simulink model "sim_dist_pos_obs_paper"  (R2020a)
settings: Solver=ode4  StartTime=0.0  StopTime=30.0  FixedStep=0.01  RelTol=1e-3
values from neighbouring files (symbols this model uses):
  alfa_theta = 20    [draw_compare_dist_pos_obs.m]
  alfa_theta_obs = 100    [draw_compare_dist_pos_obs.m]
  beta1 = 1.2    [draw_compare_dist_pos_obs.m]
  beta2 = 0.8    [draw_compare_dist_pos_obs.m]
  c1_diff_sigma_bar_v = diag([25; 30; 20])    [draw_compare_dist_pos_obs.m]
  c1v = diag([16.0; 16.0; 16.0])    [draw_compare_dist_pos_obs.m]
  c2_diff_sigma_bar_v = diag([50; 50; 10])    [draw_compare_dist_pos_obs.m]
  c2v = diag([16.0; 16.0; 16.0])    [draw_compare_dist_pos_obs.m]
  c3_diff_sigma_bar_v = diag([15; 15; 10])    [draw_compare_dist_pos_obs.m]
  c3v = diag([16.0; 16.0; 16.0])    [draw_compare_dist_pos_obs.m]
  delta_p_i_0 = zeros(3, NF)    [draw_compare_dist_pos_obs.m]
  delta_v_i_0 = zeros(3, NF)    [draw_compare_dist_pos_obs.m]
  dp_aa_t = 0.2 * ones(3, 5) + ( 1.0 - 0.2 ) * rand(3, 5)    [draw_compare_dist_pos_obs.m]
  dp_ff_t = [ 0.4 * ones(1, 5) + ( 1.0 - 0.4 ) * rand(1, 5);                      0.4 * ones(1, 5) + ( 1.0 - 0.4 ) * rand(1, 5);                      0.2 * ones(1, 5) + ( 0.6 - 0.2 ) * rand(1, 5) ]    [draw_compare_dist_pos_obs.m]
  dp_phi_t = ( - pi / 2 ) * ones(3, 5) + ( pi / 2 - ( - pi / 2 ) ) * rand(3, 5)    [draw_compare_dist_pos_obs.m]
  etai_0 = zeros(3,5)    [draw_compare_dist_pos_obs.m]
  kai_1_t = 0.02    [draw_compare_dist_pos_obs.m]
  kai_3_t = 0.1    [draw_compare_dist_pos_obs.m]
  kai_chi_1 = diag([6; 6; 6])    [draw_compare_dist_pos_obs.m]
  kai_chi_2 = diag([6; 6; 6])    [draw_compare_dist_pos_obs.m]
  kai_u_1 = diag([8; 8; 8])    [draw_compare_dist_pos_obs.m]
  kai_u_2 = diag([8; 8; 8])    [draw_compare_dist_pos_obs.m]
  ksii_0 = zeros(3,5)    [draw_compare_dist_pos_obs.m]
  l1v = diag([20; 20; 20])    [draw_compare_dist_pos_obs.m]
  l2v = diag([30; 30; 30])    [draw_compare_dist_pos_obs.m]
  Lamd_diff_sigma_bar_v = 0.5    [draw_compare_dist_pos_obs.m]
  mass_i = zeros(1,NF)    [draw_compare_dist_pos_obs.m]
  Mii = diag([1;0;0;0;1])    [draw_compare_dist_pos_obs.m]
  pos0 = zeros(3, 1)    [draw_compare_dist_pos_obs.m]
  PZ0 = P0(3)    [draw_compare_dist_pos_obs.m]
  PZ1 = 10    [draw_compare_dist_pos_obs.m]
  Qci_init = repmat([1;0;0;0],1,NF)    [draw_compare_dist_pos_obs.m]
  R0 = 4    [draw_compare_dist_pos_obs.m]
  R1 = 8    [draw_compare_dist_pos_obs.m]
  Rx2 = 10    [draw_compare_dist_pos_obs.m]
  Ry2 = 6    [draw_compare_dist_pos_obs.m]
  Rz2 = 4    [draw_compare_dist_pos_obs.m]
  T0 = 0    [draw_compare_dist_pos_obs.m]
  T1 = tseq1    (= 10)    [draw_compare_dist_pos_obs.m]
  T12 = tseq1 + tseq12    (= 20)    [draw_compare_dist_pos_obs.m]
  T2 = tseq1 + tseq12 + tseq2    (= 30)    [draw_compare_dist_pos_obs.m]
  theta0 = ( 2 / 5 ) * pi    (= 1.25663706144)    [draw_compare_dist_pos_obs.m]
  vel0 = zeros(3, 1)    [draw_compare_dist_pos_obs.m]
  Wij = [0,0,1,0,0;              0,0,1,1,0;              1,0,0,0,1;              0,1,1,0,0;              0,0,1,0,0]    [draw_compare_dist_pos_obs.m]
  X1 = 8    [draw_compare_dist_pos_obs.m]
  X2 = 2    [draw_compare_dist_pos_obs.m]
  X3 = 3    [draw_compare_dist_pos_obs.m]
  Y1 = 10    [draw_compare_dist_pos_obs.m]
  Y2 = 2    [draw_compare_dist_pos_obs.m]
  Y3 = 4    [draw_compare_dist_pos_obs.m]
  Z1 = 4    [draw_compare_dist_pos_obs.m]
  Z2 = -6    [draw_compare_dist_pos_obs.m]
  Z3 = 2    [draw_compare_dist_pos_obs.m]
  zeta_diff_sigma_bar_v = 0.08    [draw_compare_dist_pos_obs.m]
undefined symbols (not defined in the file or in its folder): cal_frac_squ, p_alfav1, p_alfav2, p_beta1, p_beta2, p_dbeta1, p_dbeta2, p_gamma1_pos, p_gamma1_vel, p_gamma2_pos, p_gamma2_vel, q_alfav1, q_alfav2, q_beta1, q_beta2, q_dbeta1, q_dbeta2, q_gamma1_pos, q_gamma1_vel, q_gamma2_pos, q_gamma2_vel
(part 2 of 5)

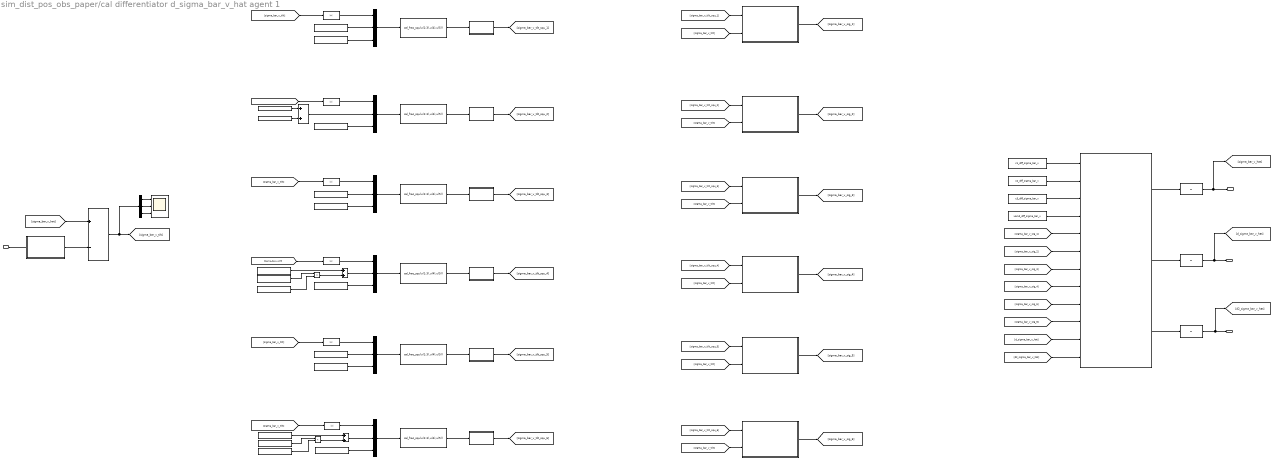
== system sim_dist_pos_obs_paper/cal differentiator d_sigma_bar_v_hat agent 1 ==
  x : Inport
  Abs{,1..5} (6 alike) : Abs
  Add : Sum
  Add1 : Sum
  Add2 : Sum
  Add3 : Sum  Inputs=+-
  Constant : Constant  Value=0
  Constant{97,100,105,107,109} (5 alike) : Constant
  Constant{98..99,101,108,110..111} (6 alike) : Constant  Value=3
  Constant102 : Constant  Value=2
  Constant103 : Constant  Value=c1_diff_sigma_bar_v
  Constant104 : Constant  Value=c2_diff_sigma_bar_v
  Constant106 : Constant  Value=c3_diff_sigma_bar_v
  Constant112 : Constant  Value=2
  Constant113 : Constant  Value=Lamd_diff_sigma_bar_v
  Constant161 : Constant  Value=zeta_diff_sigma_bar_v
  Constant162 : Constant  Value=zeta_diff_sigma_bar_v
  Constant163 : Constant  Value=zeta_diff_sigma_bar_v
  Demux2 : Demux  Outputs=3
  Integrator2 : Integrator  InitialCondition=zeros(3,1)
  Integrator3 : Integrator  InitialCondition=zeros(3,1)
  Integrator4 : Integrator  InitialCondition=zeros(3,1)
  Interpreted MATLAB Function{,20..24} (6 alike) : MATLABFcn  MATLABFcn=cal_frac_squ(u(1:3),u(4),u(5))
  Mux{19..24} (6 alike) : Mux  Inputs=3
  Product : Product
  Product1 : Product
  cal differentiator : MATLAB Function  TreatAsAtomicUnit=on
  cal sig : MATLAB Function  TreatAsAtomicUnit=on
  cal sig1 : MATLAB Function  TreatAsAtomicUnit=on
  cal sig2 : MATLAB Function  TreatAsAtomicUnit=on
  cal sig3 : MATLAB Function  TreatAsAtomicUnit=on
  cal sig4 : MATLAB Function  TreatAsAtomicUnit=on
  cal sig5 : MATLAB Function  TreatAsAtomicUnit=on
  choose sigma_bar_v : MATLAB Function  TreatAsAtomicUnit=on
  sigma_bar_v_tilt : Scope  NumInputPorts=3
  trans to column20 : MATLAB Function  TreatAsAtomicUnit=on
  trans to column21 : MATLAB Function  TreatAsAtomicUnit=on
  trans to column22 : MATLAB Function  TreatAsAtomicUnit=on
  trans to column23 : MATLAB Function  TreatAsAtomicUnit=on
  trans to column24 : MATLAB Function  TreatAsAtomicUnit=on
  trans to column25 : MATLAB Function  TreatAsAtomicUnit=on
  Out1 : Outport
  Out2 : Outport  Port=2
  Out3 : Outport  Port=3
  wires:
  Abs/1 -> Mux22/1
  [sigma_bar_v_tilt] -> cal sig/2(y)
  cal sig1/1(z) -> [sigma_bar_v_sig_2]
  [d2_sigma_bar_v_hat] -> cal differentiator/12(d2_sigma_bar_v_hat)
  trans to column23/1(y) -> [sigma_bar_v_tilt_squ_3]
  Add/1 -> Mux21/2
  Demux2/1 -> sigma_bar_v_tilt/1
  [sigma_bar_v_tilt] -> cal sig4/2(y)
  Product1/1 -> Add2/2
  Add2/1 -> Mux19/2
  [d_sigma_bar_v_hat] -> cal differentiator/11("d_sigma_bar_v_hat ")
  [sigma_bar_v_sig_3] -> cal differentiator/7(sigma_bar_v_sig_3)
  trans to column24/1(y) -> [sigma_bar_v_tilt_squ_4]
  Constant107/1 -> Mux21/3
  [sigma_bar_v_sig_5] -> cal differentiator/9(sigma_bar_v_sig_5)
  Constant97/1 -> Mux22/3
  cal sig/1(z) -> [sigma_bar_v_sig_1]
  trans to column22/1(y) -> [sigma_bar_v_tilt_squ_1]
  [sigma_bar_v_tilt_squ_3] -> cal sig2/1(x)
  [sigma_bar_v_tilt] -> Abs3/1
  Interpreted MATLAB Function24/1 -> trans to column25/1(x)
  [sigma_bar_v_sig_1] -> cal differentiator/5(sigma_bar_v_sig_1)
  cal differentiator/1(d_sigma_bar_v_hat) -> Integrator2/1
  Constant110/1 -> Mux24/3
  cal sig5/1(z) -> [sigma_bar_v_sig_5]
  [sigma_bar_v_tilt] -> Abs4/1
  Demux2/3 -> sigma_bar_v_tilt/3
  cal sig2/1(z) -> [sigma_bar_v_sig_3]
  Constant112/1 -> Product/1
  Constant/1 -> Mux22/2
  cal differentiator/3(d_d2sigma_bar_v_hat) -> Integrator4/1
  Abs3/1 -> Mux24/1
  trans to column21/1(y) -> [sigma_bar_v_tilt_squ_2]
  Constant99/1 -> Add2/1
  Constant103/1 -> cal differentiator/1(c1)
  Mux19/1 -> Interpreted MATLAB Function24/1
  [sigma_bar_v_tilt_squ_6] -> cal sig3/1(x)
  Constant106/1 -> cal differentiator/3(c3)
  [sigma_bar_v_tilt] -> Abs2/1
  [sigma_bar_v_tilt_squ_2] -> cal sig1/1(x)
  Constant162/1 -> Product/2
  Product/1 -> Add1/2
  [sigma_bar_v_sig_4] -> cal differentiator/8(sigma_bar_v_sig_4)
  [sigma_bar_v_hat] -> Add3/1
  Constant102/1 -> Mux20/2
  Add3/1 -> Demux2/1, [sigma_bar_v_tilt]
  cal differentiator/2(d_dsigma_bar_v_hat) -> Integrator3/1
  [sigma_bar_v_tilt] -> Abs5/1
  [sigma_bar_v_tilt] -> cal sig2/2(y)
  [sigma_bar_v_sig_6] -> cal differentiator/10(sigma_bar_v_sig_6)
  trans to column20/1(y) -> [sigma_bar_v_tilt_squ_5]
  Constant104/1 -> cal differentiator/2(c2)
  Constant101/1 -> Mux20/3
  Mux22/1 -> Interpreted MATLAB Function/1
  Constant163/1 -> Product1/2
  Abs2/1 -> Mux23/1
  Interpreted MATLAB Function21/1 -> trans to column21/1(x)
  Interpreted MATLAB Function23/1 -> trans to column24/1(x)
  Mux23/1 -> Interpreted MATLAB Function22/1
  cal sig3/1(z) -> [sigma_bar_v_sig_6]
  Abs4/1 -> Mux19/1
  trans to column25/1(y) -> [sigma_bar_v_tilt_squ_6]
  Constant113/1 -> cal differentiator/4(chi_t)
  choose sigma_bar_v/1(y) -> Add3/2
  Interpreted MATLAB Function/1 -> trans to column22/1(x)
  Interpreted MATLAB Function20/1 -> trans to column20/1(x)
  Constant108/1 -> Mux23/3
  [sigma_bar_v_sig_2] -> cal differentiator/6(sigma_bar_v_sig_2)
  [sigma_bar_v_tilt] -> cal sig1/2(y)
  [sigma_bar_v_tilt_squ_1] -> cal sig/1(x)
  Constant100/1 -> Product1/1
  Abs1/1 -> Mux21/1
  Demux2/2 -> sigma_bar_v_tilt/2
  Integrator4/1 -> [d2_sigma_bar_v_hat], Out3/1
  [sigma_bar_v_tilt_squ_4] -> cal sig4/1(x)
  Abs5/1 -> Mux20/1
  Constant98/1 -> Mux19/3
  Constant111/1 -> Add1/1
  [sigma_bar_v_tilt] -> cal sig5/2(y)
  Constant109/1 -> Mux23/2
  [sigma_bar_v_tilt] -> Abs/1
  Mux24/1 -> Interpreted MATLAB Function23/1
  [sigma_bar_v_tilt] -> Abs1/1
  [sigma_bar_v_tilt_squ_5] -> cal sig5/1(x)
  Add1/1 -> Mux24/2
  cal sig4/1(z) -> [sigma_bar_v_sig_4]
  Constant161/1 -> Add/2
  [sigma_bar_v_tilt] -> cal sig3/2(y)
  Mux21/1 -> Interpreted MATLAB Function21/1
  Interpreted MATLAB Function22/1 -> trans to column23/1(x)
  Mux20/1 -> Interpreted MATLAB Function20/1
  x/1 -> choose sigma_bar_v/1(x)
  Constant105/1 -> Add/1
  Integrator2/1 -> [sigma_bar_v_hat], Out1/1
  Integrator3/1 -> [d_sigma_bar_v_hat], Out2/1

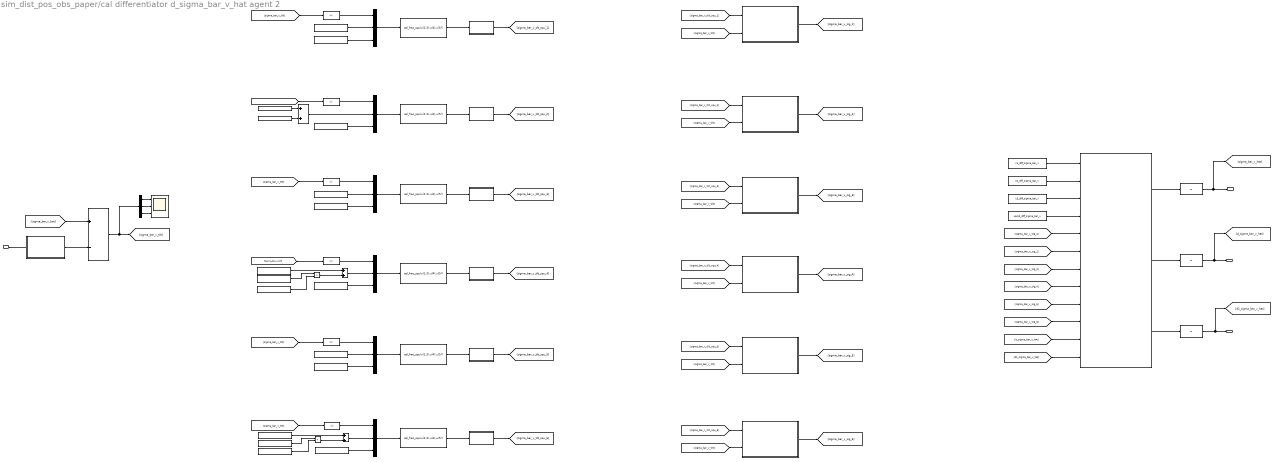
== system sim_dist_pos_obs_paper/cal differentiator d_sigma_bar_v_hat agent 2 ==
  x : Inport
  Abs{,1..5} (6 alike) : Abs
  Add : Sum
  Add1 : Sum
  Add2 : Sum
  Add3 : Sum  Inputs=+-
  Constant : Constant  Value=0
  Constant{97,100,105,107,109} (5 alike) : Constant
  Constant{98..99,101,108,110..111} (6 alike) : Constant  Value=3
  Constant102 : Constant  Value=2
  Constant103 : Constant  Value=c1_diff_sigma_bar_v
  Constant104 : Constant  Value=c2_diff_sigma_bar_v
  Constant106 : Constant  Value=c3_diff_sigma_bar_v
  Constant112 : Constant  Value=2
  Constant113 : Constant  Value=Lamd_diff_sigma_bar_v
  Constant161 : Constant  Value=zeta_diff_sigma_bar_v
  Constant162 : Constant  Value=zeta_diff_sigma_bar_v
  Constant163 : Constant  Value=zeta_diff_sigma_bar_v
  Demux2 : Demux  Outputs=3
  Integrator2 : Integrator  InitialCondition=zeros(3,1)
  Integrator3 : Integrator  InitialCondition=zeros(3,1)
  Integrator4 : Integrator  InitialCondition=zeros(3,1)
  Interpreted MATLAB Function{,20..24} (6 alike) : MATLABFcn  MATLABFcn=cal_frac_squ(u(1:3),u(4),u(5))
  Mux{19..24} (6 alike) : Mux  Inputs=3
  Product : Product
  Product1 : Product
  cal differentiator : MATLAB Function  TreatAsAtomicUnit=on
  cal sig : MATLAB Function  TreatAsAtomicUnit=on
  cal sig1 : MATLAB Function  TreatAsAtomicUnit=on
  cal sig2 : MATLAB Function  TreatAsAtomicUnit=on
  cal sig3 : MATLAB Function  TreatAsAtomicUnit=on
  cal sig4 : MATLAB Function  TreatAsAtomicUnit=on
  cal sig5 : MATLAB Function  TreatAsAtomicUnit=on
  choose sigma_bar_v : MATLAB Function  TreatAsAtomicUnit=on
  sigma_bar_v_tilt : Scope  NumInputPorts=3
  trans to column20 : MATLAB Function  TreatAsAtomicUnit=on
  trans to column21 : MATLAB Function  TreatAsAtomicUnit=on
  trans to column22 : MATLAB Function  TreatAsAtomicUnit=on
  trans to column23 : MATLAB Function  TreatAsAtomicUnit=on
  trans to column24 : MATLAB Function  TreatAsAtomicUnit=on
  trans to column25 : MATLAB Function  TreatAsAtomicUnit=on
  Out1 : Outport
  Out2 : Outport  Port=2
  Out3 : Outport  Port=3
  wires:
  Abs/1 -> Mux22/1
  [sigma_bar_v_tilt] -> cal sig/2(y)
  cal sig1/1(z) -> [sigma_bar_v_sig_2]
  [d2_sigma_bar_v_hat] -> cal differentiator/12(d2_sigma_bar_v_hat)
  trans to column23/1(y) -> [sigma_bar_v_tilt_squ_3]
  Add/1 -> Mux21/2
  Demux2/1 -> sigma_bar_v_tilt/1
  [sigma_bar_v_tilt] -> cal sig4/2(y)
  Product1/1 -> Add2/2
  Add2/1 -> Mux19/2
  [d_sigma_bar_v_hat] -> cal differentiator/11("d_sigma_bar_v_hat ")
  [sigma_bar_v_sig_3] -> cal differentiator/7(sigma_bar_v_sig_3)
  trans to column24/1(y) -> [sigma_bar_v_tilt_squ_4]
  Constant107/1 -> Mux21/3
  [sigma_bar_v_sig_5] -> cal differentiator/9(sigma_bar_v_sig_5)
  Constant97/1 -> Mux22/3
  cal sig/1(z) -> [sigma_bar_v_sig_1]
  trans to column22/1(y) -> [sigma_bar_v_tilt_squ_1]
  [sigma_bar_v_tilt_squ_3] -> cal sig2/1(x)
  [sigma_bar_v_tilt] -> Abs3/1
  Interpreted MATLAB Function24/1 -> trans to column25/1(x)
  [sigma_bar_v_sig_1] -> cal differentiator/5(sigma_bar_v_sig_1)
  cal differentiator/1(d_sigma_bar_v_hat) -> Integrator2/1
  Constant110/1 -> Mux24/3
  cal sig5/1(z) -> [sigma_bar_v_sig_5]
  [sigma_bar_v_tilt] -> Abs4/1
  Demux2/3 -> sigma_bar_v_tilt/3
  cal sig2/1(z) -> [sigma_bar_v_sig_3]
  Constant112/1 -> Product/1
  Constant/1 -> Mux22/2
  cal differentiator/3(d_d2sigma_bar_v_hat) -> Integrator4/1
  Abs3/1 -> Mux24/1
  trans to column21/1(y) -> [sigma_bar_v_tilt_squ_2]
  Constant99/1 -> Add2/1
  Constant103/1 -> cal differentiator/1(c1)
  Mux19/1 -> Interpreted MATLAB Function24/1
  [sigma_bar_v_tilt_squ_6] -> cal sig3/1(x)
  Constant106/1 -> cal differentiator/3(c3)
  [sigma_bar_v_tilt] -> Abs2/1
  [sigma_bar_v_tilt_squ_2] -> cal sig1/1(x)
  Constant162/1 -> Product/2
  Product/1 -> Add1/2
  [sigma_bar_v_sig_4] -> cal differentiator/8(sigma_bar_v_sig_4)
  [sigma_bar_v_hat] -> Add3/1
  Constant102/1 -> Mux20/2
  Add3/1 -> Demux2/1, [sigma_bar_v_tilt]
  cal differentiator/2(d_dsigma_bar_v_hat) -> Integrator3/1
  [sigma_bar_v_tilt] -> Abs5/1
  [sigma_bar_v_tilt] -> cal sig2/2(y)
  [sigma_bar_v_sig_6] -> cal differentiator/10(sigma_bar_v_sig_6)
  trans to column20/1(y) -> [sigma_bar_v_tilt_squ_5]
  Constant104/1 -> cal differentiator/2(c2)
  Constant101/1 -> Mux20/3
  Mux22/1 -> Interpreted MATLAB Function/1
  Constant163/1 -> Product1/2
  Abs2/1 -> Mux23/1
  Interpreted MATLAB Function21/1 -> trans to column21/1(x)
  Interpreted MATLAB Function23/1 -> trans to column24/1(x)
  Mux23/1 -> Interpreted MATLAB Function22/1
  cal sig3/1(z) -> [sigma_bar_v_sig_6]
  Abs4/1 -> Mux19/1
  trans to column25/1(y) -> [sigma_bar_v_tilt_squ_6]
  Constant113/1 -> cal differentiator/4(chi_t)
  choose sigma_bar_v/1(y) -> Add3/2
  Interpreted MATLAB Function/1 -> trans to column22/1(x)
  Interpreted MATLAB Function20/1 -> trans to column20/1(x)
  Constant108/1 -> Mux23/3
  [sigma_bar_v_sig_2] -> cal differentiator/6(sigma_bar_v_sig_2)
  [sigma_bar_v_tilt] -> cal sig1/2(y)
  [sigma_bar_v_tilt_squ_1] -> cal sig/1(x)
  Constant100/1 -> Product1/1
  Abs1/1 -> Mux21/1
  Demux2/2 -> sigma_bar_v_tilt/2
  Integrator4/1 -> [d2_sigma_bar_v_hat], Out3/1
  [sigma_bar_v_tilt_squ_4] -> cal sig4/1(x)
  Abs5/1 -> Mux20/1
  Constant98/1 -> Mux19/3
  Constant111/1 -> Add1/1
  [sigma_bar_v_tilt] -> cal sig5/2(y)
  Constant109/1 -> Mux23/2
  [sigma_bar_v_tilt] -> Abs/1
  Mux24/1 -> Interpreted MATLAB Function23/1
  [sigma_bar_v_tilt] -> Abs1/1
  [sigma_bar_v_tilt_squ_5] -> cal sig5/1(x)
  Add1/1 -> Mux24/2
  cal sig4/1(z) -> [sigma_bar_v_sig_4]
  Constant161/1 -> Add/2
  [sigma_bar_v_tilt] -> cal sig3/2(y)
  Mux21/1 -> Interpreted MATLAB Function21/1
  Interpreted MATLAB Function22/1 -> trans to column23/1(x)
  Mux20/1 -> Interpreted MATLAB Function20/1
  x/1 -> choose sigma_bar_v/1(x)
  Constant105/1 -> Add/1
  Integrator2/1 -> [sigma_bar_v_hat], Out1/1
  Integrator3/1 -> [d_sigma_bar_v_hat], Out2/1

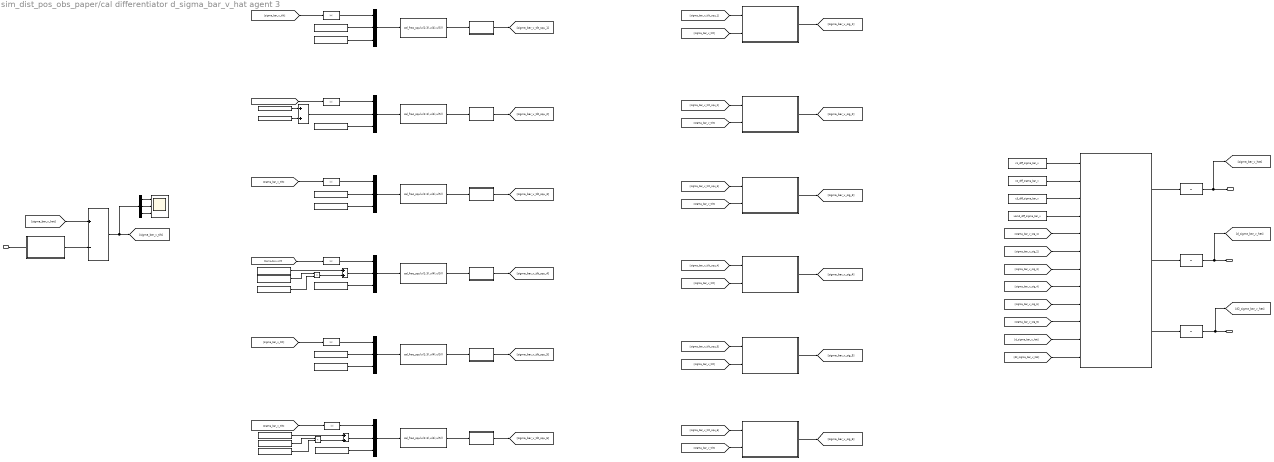
== system sim_dist_pos_obs_paper/cal differentiator d_sigma_bar_v_hat agent 3 ==
  x : Inport
  Abs{,1..5} (6 alike) : Abs
  Add : Sum
  Add1 : Sum
  Add2 : Sum
  Add3 : Sum  Inputs=+-
  Constant : Constant  Value=0
  Constant{97,100,105,107,109} (5 alike) : Constant
  Constant{98..99,101,108,110..111} (6 alike) : Constant  Value=3
  Constant102 : Constant  Value=2
  Constant103 : Constant  Value=c1_diff_sigma_bar_v
  Constant104 : Constant  Value=c2_diff_sigma_bar_v
  Constant106 : Constant  Value=c3_diff_sigma_bar_v
  Constant112 : Constant  Value=2
  Constant113 : Constant  Value=Lamd_diff_sigma_bar_v
  Constant161 : Constant  Value=zeta_diff_sigma_bar_v
  Constant162 : Constant  Value=zeta_diff_sigma_bar_v
  Constant163 : Constant  Value=zeta_diff_sigma_bar_v
  Demux2 : Demux  Outputs=3
  Integrator2 : Integrator  InitialCondition=zeros(3,1)
  Integrator3 : Integrator  InitialCondition=zeros(3,1)
  Integrator4 : Integrator  InitialCondition=zeros(3,1)
  Interpreted MATLAB Function{,20..24} (6 alike) : MATLABFcn  MATLABFcn=cal_frac_squ(u(1:3),u(4),u(5))
  Mux{19..24} (6 alike) : Mux  Inputs=3
  Product : Product
  Product1 : Product
  cal differentiator : MATLAB Function  TreatAsAtomicUnit=on
  cal sig : MATLAB Function  TreatAsAtomicUnit=on
  cal sig1 : MATLAB Function  TreatAsAtomicUnit=on
  cal sig2 : MATLAB Function  TreatAsAtomicUnit=on
  cal sig3 : MATLAB Function  TreatAsAtomicUnit=on
  cal sig4 : MATLAB Function  TreatAsAtomicUnit=on
  cal sig5 : MATLAB Function  TreatAsAtomicUnit=on
  choose sigma_bar_v : MATLAB Function  TreatAsAtomicUnit=on
  sigma_bar_v_tilt : Scope  NumInputPorts=3
  trans to column20 : MATLAB Function  TreatAsAtomicUnit=on
  trans to column21 : MATLAB Function  TreatAsAtomicUnit=on
  trans to column22 : MATLAB Function  TreatAsAtomicUnit=on
  trans to column23 : MATLAB Function  TreatAsAtomicUnit=on
  trans to column24 : MATLAB Function  TreatAsAtomicUnit=on
  trans to column25 : MATLAB Function  TreatAsAtomicUnit=on
  Out1 : Outport
  Out2 : Outport  Port=2
  Out3 : Outport  Port=3
  wires:
  Abs/1 -> Mux22/1
  [sigma_bar_v_tilt] -> cal sig/2(y)
  cal sig1/1(z) -> [sigma_bar_v_sig_2]
  [d2_sigma_bar_v_hat] -> cal differentiator/12(d2_sigma_bar_v_hat)
  trans to column23/1(y) -> [sigma_bar_v_tilt_squ_3]
  Add/1 -> Mux21/2
  Demux2/1 -> sigma_bar_v_tilt/1
  [sigma_bar_v_tilt] -> cal sig4/2(y)
  Product1/1 -> Add2/2
  Add2/1 -> Mux19/2
  [d_sigma_bar_v_hat] -> cal differentiator/11("d_sigma_bar_v_hat ")
  [sigma_bar_v_sig_3] -> cal differentiator/7(sigma_bar_v_sig_3)
  trans to column24/1(y) -> [sigma_bar_v_tilt_squ_4]
  Constant107/1 -> Mux21/3
  [sigma_bar_v_sig_5] -> cal differentiator/9(sigma_bar_v_sig_5)
  Constant97/1 -> Mux22/3
  cal sig/1(z) -> [sigma_bar_v_sig_1]
  trans to column22/1(y) -> [sigma_bar_v_tilt_squ_1]
  [sigma_bar_v_tilt_squ_3] -> cal sig2/1(x)
  [sigma_bar_v_tilt] -> Abs3/1
  Interpreted MATLAB Function24/1 -> trans to column25/1(x)
  [sigma_bar_v_sig_1] -> cal differentiator/5(sigma_bar_v_sig_1)
  cal differentiator/1(d_sigma_bar_v_hat) -> Integrator2/1
  Constant110/1 -> Mux24/3
  cal sig5/1(z) -> [sigma_bar_v_sig_5]
  [sigma_bar_v_tilt] -> Abs4/1
  Demux2/3 -> sigma_bar_v_tilt/3
  cal sig2/1(z) -> [sigma_bar_v_sig_3]
  Constant112/1 -> Product/1
  Constant/1 -> Mux22/2
  cal differentiator/3(d_d2sigma_bar_v_hat) -> Integrator4/1
  Abs3/1 -> Mux24/1
  trans to column21/1(y) -> [sigma_bar_v_tilt_squ_2]
  Constant99/1 -> Add2/1
  Constant103/1 -> cal differentiator/1(c1)
  Mux19/1 -> Interpreted MATLAB Function24/1
  [sigma_bar_v_tilt_squ_6] -> cal sig3/1(x)
  Constant106/1 -> cal differentiator/3(c3)
  [sigma_bar_v_tilt] -> Abs2/1
  [sigma_bar_v_tilt_squ_2] -> cal sig1/1(x)
  Constant162/1 -> Product/2
  Product/1 -> Add1/2
  [sigma_bar_v_sig_4] -> cal differentiator/8(sigma_bar_v_sig_4)
  [sigma_bar_v_hat] -> Add3/1
  Constant102/1 -> Mux20/2
  Add3/1 -> Demux2/1, [sigma_bar_v_tilt]
  cal differentiator/2(d_dsigma_bar_v_hat) -> Integrator3/1
  [sigma_bar_v_tilt] -> Abs5/1
  [sigma_bar_v_tilt] -> cal sig2/2(y)
  [sigma_bar_v_sig_6] -> cal differentiator/10(sigma_bar_v_sig_6)
  trans to column20/1(y) -> [sigma_bar_v_tilt_squ_5]
  Constant104/1 -> cal differentiator/2(c2)
  Constant101/1 -> Mux20/3
  Mux22/1 -> Interpreted MATLAB Function/1
  Constant163/1 -> Product1/2
  Abs2/1 -> Mux23/1
  Interpreted MATLAB Function21/1 -> trans to column21/1(x)
  Interpreted MATLAB Function23/1 -> trans to column24/1(x)
  Mux23/1 -> Interpreted MATLAB Function22/1
  cal sig3/1(z) -> [sigma_bar_v_sig_6]
  Abs4/1 -> Mux19/1
  trans to column25/1(y) -> [sigma_bar_v_tilt_squ_6]
  Constant113/1 -> cal differentiator/4(chi_t)
  choose sigma_bar_v/1(y) -> Add3/2
  Interpreted MATLAB Function/1 -> trans to column22/1(x)
  Interpreted MATLAB Function20/1 -> trans to column20/1(x)
  Constant108/1 -> Mux23/3
  [sigma_bar_v_sig_2] -> cal differentiator/6(sigma_bar_v_sig_2)
  [sigma_bar_v_tilt] -> cal sig1/2(y)
  [sigma_bar_v_tilt_squ_1] -> cal sig/1(x)
  Constant100/1 -> Product1/1
  Abs1/1 -> Mux21/1
  Demux2/2 -> sigma_bar_v_tilt/2
  Integrator4/1 -> [d2_sigma_bar_v_hat], Out3/1
  [sigma_bar_v_tilt_squ_4] -> cal sig4/1(x)
  Abs5/1 -> Mux20/1
  Constant98/1 -> Mux19/3
  Constant111/1 -> Add1/1
  [sigma_bar_v_tilt] -> cal sig5/2(y)
  Constant109/1 -> Mux23/2
  [sigma_bar_v_tilt] -> Abs/1
  Mux24/1 -> Interpreted MATLAB Function23/1
  [sigma_bar_v_tilt] -> Abs1/1
  [sigma_bar_v_tilt_squ_5] -> cal sig5/1(x)
  Add1/1 -> Mux24/2
  cal sig4/1(z) -> [sigma_bar_v_sig_4]
  Constant161/1 -> Add/2
  [sigma_bar_v_tilt] -> cal sig3/2(y)
  Mux21/1 -> Interpreted MATLAB Function21/1
  Interpreted MATLAB Function22/1 -> trans to column23/1(x)
  Mux20/1 -> Interpreted MATLAB Function20/1
  x/1 -> choose sigma_bar_v/1(x)
  Constant105/1 -> Add/1
  Integrator2/1 -> [sigma_bar_v_hat], Out1/1
  Integrator3/1 -> [d_sigma_bar_v_hat], Out2/1

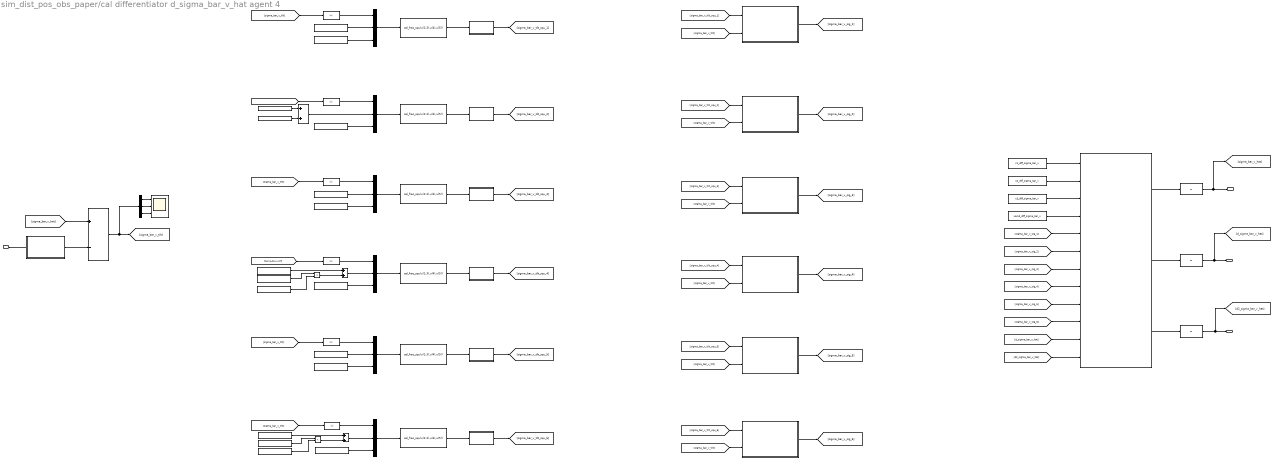
== system sim_dist_pos_obs_paper/cal differentiator d_sigma_bar_v_hat agent 4 ==
  x : Inport
  Abs{,1..5} (6 alike) : Abs
  Add : Sum
  Add1 : Sum
  Add2 : Sum
  Add3 : Sum  Inputs=+-
  Constant : Constant  Value=0
  Constant{97,100,105,107,109} (5 alike) : Constant
  Constant{98..99,101,108,110..111} (6 alike) : Constant  Value=3
  Constant102 : Constant  Value=2
  Constant103 : Constant  Value=c1_diff_sigma_bar_v
  Constant104 : Constant  Value=c2_diff_sigma_bar_v
  Constant106 : Constant  Value=c3_diff_sigma_bar_v
  Constant112 : Constant  Value=2
  Constant113 : Constant  Value=Lamd_diff_sigma_bar_v
  Constant161 : Constant  Value=zeta_diff_sigma_bar_v
  Constant162 : Constant  Value=zeta_diff_sigma_bar_v
  Constant163 : Constant  Value=zeta_diff_sigma_bar_v
  Demux2 : Demux  Outputs=3
  Integrator2 : Integrator  InitialCondition=zeros(3,1)
  Integrator3 : Integrator  InitialCondition=zeros(3,1)
  Integrator4 : Integrator  InitialCondition=zeros(3,1)
  Interpreted MATLAB Function{,20..24} (6 alike) : MATLABFcn  MATLABFcn=cal_frac_squ(u(1:3),u(4),u(5))
  Mux{19..24} (6 alike) : Mux  Inputs=3
  Product : Product
  Product1 : Product
  cal differentiator : MATLAB Function  TreatAsAtomicUnit=on
  cal sig : MATLAB Function  TreatAsAtomicUnit=on
  cal sig1 : MATLAB Function  TreatAsAtomicUnit=on
  cal sig2 : MATLAB Function  TreatAsAtomicUnit=on
  cal sig3 : MATLAB Function  TreatAsAtomicUnit=on
  cal sig4 : MATLAB Function  TreatAsAtomicUnit=on
  cal sig5 : MATLAB Function  TreatAsAtomicUnit=on
  choose sigma_bar_v : MATLAB Function  TreatAsAtomicUnit=on
  sigma_bar_v_tilt : Scope  NumInputPorts=3
  trans to column20 : MATLAB Function  TreatAsAtomicUnit=on
  trans to column21 : MATLAB Function  TreatAsAtomicUnit=on
  trans to column22 : MATLAB Function  TreatAsAtomicUnit=on
  trans to column23 : MATLAB Function  TreatAsAtomicUnit=on
  trans to column24 : MATLAB Function  TreatAsAtomicUnit=on
  trans to column25 : MATLAB Function  TreatAsAtomicUnit=on
  Out1 : Outport
  Out2 : Outport  Port=2
  Out3 : Outport  Port=3
  wires:
  Abs/1 -> Mux22/1
  [sigma_bar_v_tilt] -> cal sig/2(y)
  cal sig1/1(z) -> [sigma_bar_v_sig_2]
  [d2_sigma_bar_v_hat] -> cal differentiator/12(d2_sigma_bar_v_hat)
  trans to column23/1(y) -> [sigma_bar_v_tilt_squ_3]
  Add/1 -> Mux21/2
  Demux2/1 -> sigma_bar_v_tilt/1
  [sigma_bar_v_tilt] -> cal sig4/2(y)
  Product1/1 -> Add2/2
  Add2/1 -> Mux19/2
  [d_sigma_bar_v_hat] -> cal differentiator/11("d_sigma_bar_v_hat ")
  [sigma_bar_v_sig_3] -> cal differentiator/7(sigma_bar_v_sig_3)
  trans to column24/1(y) -> [sigma_bar_v_tilt_squ_4]
  Constant107/1 -> Mux21/3
  [sigma_bar_v_sig_5] -> cal differentiator/9(sigma_bar_v_sig_5)
  Constant97/1 -> Mux22/3
  cal sig/1(z) -> [sigma_bar_v_sig_1]
  trans to column22/1(y) -> [sigma_bar_v_tilt_squ_1]
  [sigma_bar_v_tilt_squ_3] -> cal sig2/1(x)
  [sigma_bar_v_tilt] -> Abs3/1
  Interpreted MATLAB Function24/1 -> trans to column25/1(x)
  [sigma_bar_v_sig_1] -> cal differentiator/5(sigma_bar_v_sig_1)
  cal differentiator/1(d_sigma_bar_v_hat) -> Integrator2/1
  Constant110/1 -> Mux24/3
  cal sig5/1(z) -> [sigma_bar_v_sig_5]
  [sigma_bar_v_tilt] -> Abs4/1
  Demux2/3 -> sigma_bar_v_tilt/3
  cal sig2/1(z) -> [sigma_bar_v_sig_3]
  Constant112/1 -> Product/1
  Constant/1 -> Mux22/2
  cal differentiator/3(d_d2sigma_bar_v_hat) -> Integrator4/1
  Abs3/1 -> Mux24/1
  trans to column21/1(y) -> [sigma_bar_v_tilt_squ_2]
  Constant99/1 -> Add2/1
  Constant103/1 -> cal differentiator/1(c1)
  Mux19/1 -> Interpreted MATLAB Function24/1
  [sigma_bar_v_tilt_squ_6] -> cal sig3/1(x)
  Constant106/1 -> cal differentiator/3(c3)
  [sigma_bar_v_tilt] -> Abs2/1
  [sigma_bar_v_tilt_squ_2] -> cal sig1/1(x)
  Constant162/1 -> Product/2
  Product/1 -> Add1/2
  [sigma_bar_v_sig_4] -> cal differentiator/8(sigma_bar_v_sig_4)
  [sigma_bar_v_hat] -> Add3/1
  Constant102/1 -> Mux20/2
  Add3/1 -> Demux2/1, [sigma_bar_v_tilt]
  cal differentiator/2(d_dsigma_bar_v_hat) -> Integrator3/1
  [sigma_bar_v_tilt] -> Abs5/1
  [sigma_bar_v_tilt] -> cal sig2/2(y)
  [sigma_bar_v_sig_6] -> cal differentiator/10(sigma_bar_v_sig_6)
  trans to column20/1(y) -> [sigma_bar_v_tilt_squ_5]
  Constant104/1 -> cal differentiator/2(c2)
  Constant101/1 -> Mux20/3
  Mux22/1 -> Interpreted MATLAB Function/1
  Constant163/1 -> Product1/2
  Abs2/1 -> Mux23/1
  Interpreted MATLAB Function21/1 -> trans to column21/1(x)
  Interpreted MATLAB Function23/1 -> trans to column24/1(x)
  Mux23/1 -> Interpreted MATLAB Function22/1
  cal sig3/1(z) -> [sigma_bar_v_sig_6]
  Abs4/1 -> Mux19/1
  trans to column25/1(y) -> [sigma_bar_v_tilt_squ_6]
  Constant113/1 -> cal differentiator/4(chi_t)
  choose sigma_bar_v/1(y) -> Add3/2
  Interpreted MATLAB Function/1 -> trans to column22/1(x)
  Interpreted MATLAB Function20/1 -> trans to column20/1(x)
  Constant108/1 -> Mux23/3
  [sigma_bar_v_sig_2] -> cal differentiator/6(sigma_bar_v_sig_2)
  [sigma_bar_v_tilt] -> cal sig1/2(y)
  [sigma_bar_v_tilt_squ_1] -> cal sig/1(x)
  Constant100/1 -> Product1/1
  Abs1/1 -> Mux21/1
  Demux2/2 -> sigma_bar_v_tilt/2
  Integrator4/1 -> [d2_sigma_bar_v_hat], Out3/1
  [sigma_bar_v_tilt_squ_4] -> cal sig4/1(x)
  Abs5/1 -> Mux20/1
  Constant98/1 -> Mux19/3
  Constant111/1 -> Add1/1
  [sigma_bar_v_tilt] -> cal sig5/2(y)
  Constant109/1 -> Mux23/2
  [sigma_bar_v_tilt] -> Abs/1
  Mux24/1 -> Interpreted MATLAB Function23/1
  [sigma_bar_v_tilt] -> Abs1/1
  [sigma_bar_v_tilt_squ_5] -> cal sig5/1(x)
  Add1/1 -> Mux24/2
  cal sig4/1(z) -> [sigma_bar_v_sig_4]
  Constant161/1 -> Add/2
  [sigma_bar_v_tilt] -> cal sig3/2(y)
  Mux21/1 -> Interpreted MATLAB Function21/1
  Interpreted MATLAB Function22/1 -> trans to column23/1(x)
  Mux20/1 -> Interpreted MATLAB Function20/1
  x/1 -> choose sigma_bar_v/1(x)
  Constant105/1 -> Add/1
  Integrator2/1 -> [sigma_bar_v_hat], Out1/1
  Integrator3/1 -> [d_sigma_bar_v_hat], Out2/1

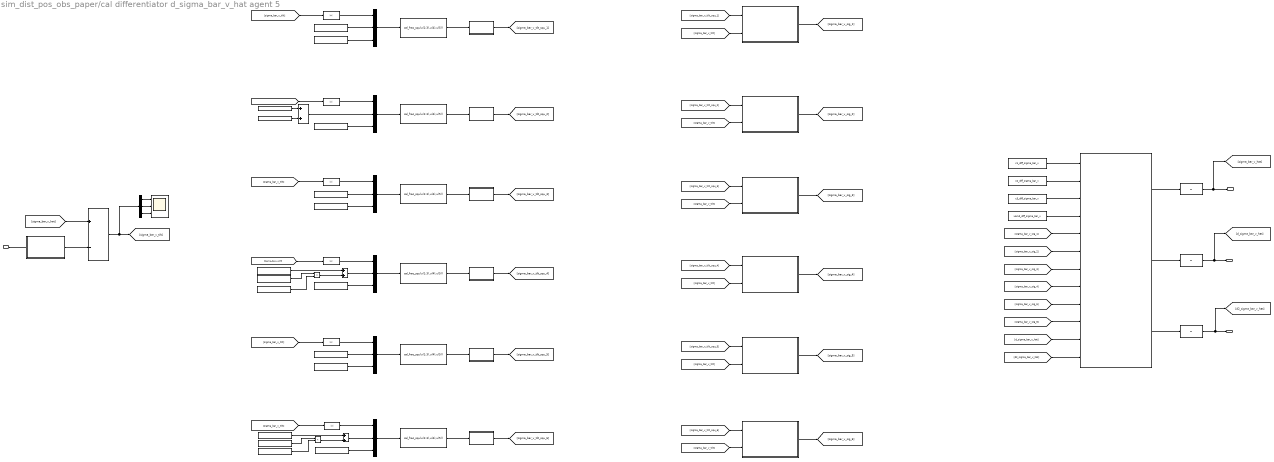
== system sim_dist_pos_obs_paper/cal differentiator d_sigma_bar_v_hat agent 5 ==
  x : Inport
  Abs{,1..5} (6 alike) : Abs
  Add : Sum
  Add1 : Sum
  Add2 : Sum
  Add3 : Sum  Inputs=+-
  Constant : Constant  Value=0
  Constant{97,100,105,107,109} (5 alike) : Constant
  Constant{98..99,101,108,110..111} (6 alike) : Constant  Value=3
  Constant102 : Constant  Value=2
  Constant103 : Constant  Value=c1_diff_sigma_bar_v
  Constant104 : Constant  Value=c2_diff_sigma_bar_v
  Constant106 : Constant  Value=c3_diff_sigma_bar_v
  Constant112 : Constant  Value=2
  Constant113 : Constant  Value=Lamd_diff_sigma_bar_v
  Constant161 : Constant  Value=zeta_diff_sigma_bar_v
  Constant162 : Constant  Value=zeta_diff_sigma_bar_v
  Constant163 : Constant  Value=zeta_diff_sigma_bar_v
  Demux2 : Demux  Outputs=3
  Integrator2 : Integrator  InitialCondition=zeros(3,1)
  Integrator3 : Integrator  InitialCondition=zeros(3,1)
  Integrator4 : Integrator  InitialCondition=zeros(3,1)
  Interpreted MATLAB Function{,20..24} (6 alike) : MATLABFcn  MATLABFcn=cal_frac_squ(u(1:3),u(4),u(5))
  Mux{19..24} (6 alike) : Mux  Inputs=3
  Product : Product
  Product1 : Product
  cal differentiator : MATLAB Function  TreatAsAtomicUnit=on
  cal sig : MATLAB Function  TreatAsAtomicUnit=on
  cal sig1 : MATLAB Function  TreatAsAtomicUnit=on
  cal sig2 : MATLAB Function  TreatAsAtomicUnit=on
  cal sig3 : MATLAB Function  TreatAsAtomicUnit=on
  cal sig4 : MATLAB Function  TreatAsAtomicUnit=on
  cal sig5 : MATLAB Function  TreatAsAtomicUnit=on
  choose sigma_bar_v : MATLAB Function  TreatAsAtomicUnit=on
  sigma_bar_v_tilt : Scope  NumInputPorts=3
  trans to column20 : MATLAB Function  TreatAsAtomicUnit=on
  trans to column21 : MATLAB Function  TreatAsAtomicUnit=on
  trans to column22 : MATLAB Function  TreatAsAtomicUnit=on
  trans to column23 : MATLAB Function  TreatAsAtomicUnit=on
  trans to column24 : MATLAB Function  TreatAsAtomicUnit=on
  trans to column25 : MATLAB Function  TreatAsAtomicUnit=on
  Out1 : Outport
  Out2 : Outport  Port=2
  Out3 : Outport  Port=3
  wires:
  Abs/1 -> Mux22/1
  [sigma_bar_v_tilt] -> cal sig/2(y)
  cal sig1/1(z) -> [sigma_bar_v_sig_2]
  [d2_sigma_bar_v_hat] -> cal differentiator/12(d2_sigma_bar_v_hat)
  trans to column23/1(y) -> [sigma_bar_v_tilt_squ_3]
  Add/1 -> Mux21/2
  Demux2/1 -> sigma_bar_v_tilt/1
  [sigma_bar_v_tilt] -> cal sig4/2(y)
  Product1/1 -> Add2/2
  Add2/1 -> Mux19/2
  [d_sigma_bar_v_hat] -> cal differentiator/11("d_sigma_bar_v_hat ")
  [sigma_bar_v_sig_3] -> cal differentiator/7(sigma_bar_v_sig_3)
  trans to column24/1(y) -> [sigma_bar_v_tilt_squ_4]
  Constant107/1 -> Mux21/3
  [sigma_bar_v_sig_5] -> cal differentiator/9(sigma_bar_v_sig_5)
  Constant97/1 -> Mux22/3
  cal sig/1(z) -> [sigma_bar_v_sig_1]
  trans to column22/1(y) -> [sigma_bar_v_tilt_squ_1]
  [sigma_bar_v_tilt_squ_3] -> cal sig2/1(x)
  [sigma_bar_v_tilt] -> Abs3/1
  Interpreted MATLAB Function24/1 -> trans to column25/1(x)
  [sigma_bar_v_sig_1] -> cal differentiator/5(sigma_bar_v_sig_1)
  cal differentiator/1(d_sigma_bar_v_hat) -> Integrator2/1
  Constant110/1 -> Mux24/3
  cal sig5/1(z) -> [sigma_bar_v_sig_5]
  [sigma_bar_v_tilt] -> Abs4/1
  Demux2/3 -> sigma_bar_v_tilt/3
  cal sig2/1(z) -> [sigma_bar_v_sig_3]
  Constant112/1 -> Product/1
  Constant/1 -> Mux22/2
  cal differentiator/3(d_d2sigma_bar_v_hat) -> Integrator4/1
  Abs3/1 -> Mux24/1
  trans to column21/1(y) -> [sigma_bar_v_tilt_squ_2]
  Constant99/1 -> Add2/1
  Constant103/1 -> cal differentiator/1(c1)
  Mux19/1 -> Interpreted MATLAB Function24/1
  [sigma_bar_v_tilt_squ_6] -> cal sig3/1(x)
  Constant106/1 -> cal differentiator/3(c3)
  [sigma_bar_v_tilt] -> Abs2/1
  [sigma_bar_v_tilt_squ_2] -> cal sig1/1(x)
  Constant162/1 -> Product/2
  Product/1 -> Add1/2
  [sigma_bar_v_sig_4] -> cal differentiator/8(sigma_bar_v_sig_4)
  [sigma_bar_v_hat] -> Add3/1
  Constant102/1 -> Mux20/2
  Add3/1 -> Demux2/1, [sigma_bar_v_tilt]
  cal differentiator/2(d_dsigma_bar_v_hat) -> Integrator3/1
  [sigma_bar_v_tilt] -> Abs5/1
  [sigma_bar_v_tilt] -> cal sig2/2(y)
  [sigma_bar_v_sig_6] -> cal differentiator/10(sigma_bar_v_sig_6)
  trans to column20/1(y) -> [sigma_bar_v_tilt_squ_5]
  Constant104/1 -> cal differentiator/2(c2)
  Constant101/1 -> Mux20/3
  Mux22/1 -> Interpreted MATLAB Function/1
  Constant163/1 -> Product1/2
  Abs2/1 -> Mux23/1
  Interpreted MATLAB Function21/1 -> trans to column21/1(x)
  Interpreted MATLAB Function23/1 -> trans to column24/1(x)
  Mux23/1 -> Interpreted MATLAB Function22/1
  cal sig3/1(z) -> [sigma_bar_v_sig_6]
  Abs4/1 -> Mux19/1
  trans to column25/1(y) -> [sigma_bar_v_tilt_squ_6]
  Constant113/1 -> cal differentiator/4(chi_t)
  choose sigma_bar_v/1(y) -> Add3/2
  Interpreted MATLAB Function/1 -> trans to column22/1(x)
  Interpreted MATLAB Function20/1 -> trans to column20/1(x)
  Constant108/1 -> Mux23/3
  [sigma_bar_v_sig_2] -> cal differentiator/6(sigma_bar_v_sig_2)
  [sigma_bar_v_tilt] -> cal sig1/2(y)
  [sigma_bar_v_tilt_squ_1] -> cal sig/1(x)
  Constant100/1 -> Product1/1
  Abs1/1 -> Mux21/1
  Demux2/2 -> sigma_bar_v_tilt/2
  Integrator4/1 -> [d2_sigma_bar_v_hat], Out3/1
  [sigma_bar_v_tilt_squ_4] -> cal sig4/1(x)
  Abs5/1 -> Mux20/1
  Constant98/1 -> Mux19/3
  Constant111/1 -> Add1/1
  [sigma_bar_v_tilt] -> cal sig5/2(y)
  Constant109/1 -> Mux23/2
  [sigma_bar_v_tilt] -> Abs/1
  Mux24/1 -> Interpreted MATLAB Function23/1
  [sigma_bar_v_tilt] -> Abs1/1
  [sigma_bar_v_tilt_squ_5] -> cal sig5/1(x)
  Add1/1 -> Mux24/2
  cal sig4/1(z) -> [sigma_bar_v_sig_4]
  Constant161/1 -> Add/2
  [sigma_bar_v_tilt] -> cal sig3/2(y)
  Mux21/1 -> Interpreted MATLAB Function21/1
  Interpreted MATLAB Function22/1 -> trans to column23/1(x)
  Mux20/1 -> Interpreted MATLAB Function20/1
  x/1 -> choose sigma_bar_v/1(x)
  Constant105/1 -> Add/1
  Integrator2/1 -> [sigma_bar_v_hat], Out1/1
  Integrator3/1 -> [d_sigma_bar_v_hat], Out2/1

== matlab function sim_dist_pos_obs_paper/choose ksi_est_err 20 ==
  data: x input; y output
function y = fcn(x)
iiuav = 5;
y = x(:,iiuav);

== matlab function sim_dist_pos_obs_paper/trans to column18 ==
  data: x input; y output
function y = fcn(x)
y = x(:);

== matlab function sim_dist_pos_obs_paper/trans to column19 ==
  data: x input; y output
function y = fcn(x)
y = x(:);

== matlab function sim_dist_pos_obs_paper/cal dchi agent 1 ==
  data: kai_chi_1 input; d_chi_1 output; kai_chi_2 input; d_theta_err_ksi_1_vec input; d_theta_err_ksi_2_vec input
function d_chi_1 = fcn(kai_chi_1, kai_chi_2, d_theta_err_ksi_1_vec, d_theta_err_ksi_2_vec)
%%%% 固定时间虚拟速度控制量导数d_chi
iiuav = 1;
d_chi_1 = -kai_chi_1 * d_theta_err_ksi_1_vec(:,iiuav) - kai_chi_2 * d_theta_err_ksi_2_vec(:,iiuav);

== matlab function sim_dist_pos_obs_paper/combine dtheta_err_ksi ==
  data: d_theta_err_ksi_1_1 input; d_theta_err_ksi_1_2 input; d_theta_err_ksi_1_3 input; d_theta_err_ksi_1_4 input; d_theta_err_ksi_1_5 input; d_theta_err_ksi_1_vec output; d_theta_err_ksi_2_1 input; d_theta_err_ksi_2_vec output; d_theta_err_ksi_2_2 input; d_theta_err_ksi_2_3 input; d_theta_err_ksi_2_4 input; d_theta_err_ksi_2_5 input
function [d_theta_err_ksi_1_vec, d_theta_err_ksi_2_vec]  = fcn(d_theta_err_ksi_1_1, d_theta_err_ksi_1_2, d_theta_err_ksi_1_3, d_theta_err_ksi_1_4, d_theta_err_ksi_1_5, ...
                                                                                                                d_theta_err_ksi_2_1, d_theta_err_ksi_2_2, d_theta_err_ksi_2_3, d_theta_err_ksi_2_4, d_theta_err_ksi_2_5)
%%%% 合并平滑函数的导数
d_theta_err_ksi_1_vec = [d_theta_err_ksi_1_1(:), d_theta_err_ksi_1_2(:), d_theta_err_ksi_1_3(:), d_theta_err_ksi_1_4(:), d_theta_err_ksi_1_5(:)];
d_theta_err_ksi_2_vec = [d_theta_err_ksi_2_1(:), d_theta_err_ksi_2_2(:), d_theta_err_ksi_2_3(:), d_theta_err_ksi_2_4(:), d_theta_err_ksi_2_5(:)];

== matlab function sim_dist_pos_obs_paper/generate translational disturbance agent 4 ==
  data: dp_aa_t input; dp_ff_t input; dp_phi_t input; dp_4 output; t input
function dp_4 = fcn(dp_aa_t, dp_ff_t, dp_phi_t, t)
%%%% 平移动力学方程中的扰动项设置
epsil_t = zeros(3, 1);

for kk = 1:5
    epsil_t = epsil_t + dp_aa_t(:, kk) .* sin( 2 * pi * dp_ff_t(:, kk) * t + dp_phi_t(:, kk) );
end

dp_4 = [ epsil_t(1) + 1.6 * sin( 0.2 * t ) + 2.0 * cos( 0.3 * t ) + 1.4 * sin( 0.5 * t ) ...
                + 4 * exp( -0.1 * t ) * sin( 0.5 * t ) + 3 / ( 1 + exp( -0.2 * ( t - 15 ) ) ); ...
                epsil_t(2) + 1.2 * sin( 0.1 * t ) + 3 * cos( 0.2 * t ) + 0.8 * sin( 0.4 * t ) ...
                + 2 * exp( -0.15 * t ) * cos( 0.6 * t ) + 3 / ( 1 + exp( -0.3 * ( t - 25 ) ) ); ...
                epsil_t(3) + 1.8 * sin( 0.1 * t ) + 1.6 * sin( 0.2 * t ) + 1.6 * cos( 0.3 * t ) ...
                + 4 * exp( -0.05 * t ) * sin( 0.4 * t + pi / 4 ) + 3 / ( 1 + exp( -0.5 * ( t - 20 ) ) ) ];

== matlab function sim_dist_pos_obs_paper/cal dchi agent 2 ==
  data: kai_chi_1 input; d_chi_2 output; kai_chi_2 input; d_theta_err_ksi_1_vec input; d_theta_err_ksi_2_vec input
function d_chi_2 = fcn(kai_chi_1, kai_chi_2, d_theta_err_ksi_1_vec, d_theta_err_ksi_2_vec)
%%%% 固定时间虚拟速度控制量导数d_chi
iiuav = 2;
d_chi_2 = -kai_chi_1 * d_theta_err_ksi_1_vec(:,iiuav) - kai_chi_2 * d_theta_err_ksi_2_vec(:,iiuav);

== matlab function sim_dist_pos_obs_paper/cal dchi agent 3 ==
  data: kai_chi_1 input; d_chi_3 output; kai_chi_2 input; d_theta_err_ksi_1_vec input; d_theta_err_ksi_2_vec input
function d_chi_3 = fcn(kai_chi_1, kai_chi_2, d_theta_err_ksi_1_vec, d_theta_err_ksi_2_vec)
%%%% 固定时间虚拟速度控制量导数d_chi
iiuav = 3;
d_chi_3 = -kai_chi_1 * d_theta_err_ksi_1_vec(:,iiuav) - kai_chi_2 * d_theta_err_ksi_2_vec(:,iiuav);

== matlab function sim_dist_pos_obs_paper/cal dchi agent 4 ==
  data: kai_chi_1 input; d_chi_4 output; kai_chi_2 input; d_theta_err_ksi_1_vec input; d_theta_err_ksi_2_vec input
function d_chi_4 = fcn(kai_chi_1, kai_chi_2, d_theta_err_ksi_1_vec, d_theta_err_ksi_2_vec)
%%%% 固定时间虚拟速度控制量导数d_chi
iiuav = 4;
d_chi_4 = -kai_chi_1 * d_theta_err_ksi_1_vec(:,iiuav) - kai_chi_2 * d_theta_err_ksi_2_vec(:,iiuav);

== matlab function sim_dist_pos_obs_paper/cal dchi agent 5 ==
  data: kai_chi_1 input; d_chi_5 output; kai_chi_2 input; d_theta_err_ksi_1_vec input; d_theta_err_ksi_2_vec input
function d_chi_5 = fcn(kai_chi_1, kai_chi_2, d_theta_err_ksi_1_vec, d_theta_err_ksi_2_vec)
%%%% 固定时间虚拟速度控制量导数d_chi
iiuav = 5;
d_chi_5 = -kai_chi_1 * d_theta_err_ksi_1_vec(:,iiuav) - kai_chi_2 * d_theta_err_ksi_2_vec(:,iiuav);

== matlab function sim_dist_pos_obs_paper/combine dchi ==
  data: d_chi_1 input; d_chi_2 input; d_chi_3 input; d_chi_4 input; d_chi_5 input; d_chi_vec output
function d_chi_vec  = fcn(d_chi_1, d_chi_2, d_chi_3, d_chi_4, d_chi_5)
%%%% 合并领导者位置观测器输出结果
d_chi_vec = [d_chi_1(:), d_chi_2(:), d_chi_3(:), d_chi_4(:), d_chi_5(:)];

== matlab function sim_dist_pos_obs_paper/cal virtual control sigma_v agent 1 ==
  data: c3v input; Ri input; ui_vec input; d_sigma_v_1 output; sigma_bar_v_vec input
function d_sigma_v_1 = fcn(c3v, Ri, ui_vec, sigma_bar_v_vec)
%%%% 计算扰动观测器中虚拟速度控制量sigma_v的微分方程

iiuav = 1;
g0 = 9.80663;
e3 = [0;0;1];
d_sigma_v_1 = -g0 * e3 + norm(ui_vec(:,iiuav), 2) * Ri(:,:,iiuav) * e3 + c3v * sigma_bar_v_vec(:,iiuav);

== matlab function sim_dist_pos_obs_paper/cal virtual control sigma_v agent 2 ==
  data: c3v input; Ri input; ui_vec input; d_sigma_v_2 output; sigma_bar_v_vec input
function d_sigma_v_2 = fcn(c3v, Ri, ui_vec, sigma_bar_v_vec)
%%%% 计算扰动观测器中虚拟速度控制量sigma_v的微分方程

iiuav = 2;
g0 = 9.80663;
e3 = [0;0;1];
d_sigma_v_2 = -g0 * e3 + norm(ui_vec(:,iiuav), 2) * Ri(:,:,iiuav) * e3 + c3v * sigma_bar_v_vec(:,iiuav);

== matlab function sim_dist_pos_obs_paper/cal virtual control sigma_v agent 3 ==
  data: c3v input; Ri input; ui_vec input; d_sigma_v_3 output; sigma_bar_v_vec input
function d_sigma_v_3 = fcn(c3v, Ri, ui_vec, sigma_bar_v_vec)
%%%% 计算扰动观测器中虚拟速度控制量sigma_v的微分方程

iiuav = 3;
g0 = 9.80663;
e3 = [0;0;1];
d_sigma_v_3 = -g0 * e3 + norm(ui_vec(:,iiuav), 2) * Ri(:,:,iiuav) * e3 + c3v * sigma_bar_v_vec(:,iiuav);

== matlab function sim_dist_pos_obs_paper/cal virtual control sigma_v agent 4 ==
  data: c3v input; Ri input; ui_vec input; d_sigma_v_4 output; sigma_bar_v_vec input
function d_sigma_v_4 = fcn(c3v, Ri, ui_vec, sigma_bar_v_vec)
%%%% 计算扰动观测器中虚拟速度控制量sigma_v的微分方程

iiuav = 4;
g0 = 9.80663;
e3 = [0;0;1];
d_sigma_v_4 = -g0 * e3 + norm(ui_vec(:,iiuav), 2) * Ri(:,:,iiuav) * e3 + c3v * sigma_bar_v_vec(:,iiuav);

== matlab function sim_dist_pos_obs_paper/cal virtual control sigma_v agent 5 ==
  data: c3v input; Ri input; ui_vec input; d_sigma_v_5 output; sigma_bar_v_vec input
function d_sigma_v_5 = fcn(c3v, Ri, ui_vec, sigma_bar_v_vec)
%%%% 计算扰动观测器中虚拟速度控制量sigma_v的微分方程

iiuav = 5;
g0 = 9.80663;
e3 = [0;0;1];
d_sigma_v_5 = -g0 * e3 + norm(ui_vec(:,iiuav), 2) * Ri(:,:,iiuav) * e3 + c3v * sigma_bar_v_vec(:,iiuav);

== matlab function sim_dist_pos_obs_paper/leader control input ==
  data: t input; u0 output; T1 input; T2 input; R0 input; R1 input; Rx2 input; Ry2 input; Rz2 input
function u0  = fcn(t, T1, T2, R0, R1, Rx2, Ry2, Rz2)
%%%% 给出领导者参考加速度控制输入
u0 = zeros(3, 1);

if t <= ( T1 + 1e-05 )
    u0(1, 1) = - ( 4 * pi * sin( ( 2 * pi * ( t - 0 ) ) / ( 0 - T1 ) ) * ( R0 - R1 ) ) / ( ( 0 - T1 ) ^ 2 ) ...
                        - ( 4 * ( pi ^ 2 ) * cos( ( 2 * pi * ( t - 0 ) ) / ( 0 - T1 ) ) ...
                        * ( R0 + ( ( R0 - R1 ) * ( t - 0 ) ) / ( 0 - T1 ) ) ) / ( ( 0 - T1 ) ^ 2 );
    u0(2, 1) = ( 4 * pi * cos( ( 2 * pi * ( t - 0 ) ) / ( 0 - T1 ) ) * ( R0 - R1 ) ) / ( ( 0 - T1 ) ^ 2 ) ...
                        - ( 4 * ( pi ^ 2 ) * sin( ( 2 * pi * ( t - 0 ) ) / ( 0 - T1 ) ) ...
                        * ( R0 + ( ( R0 - R1 ) * ( t - 0 ) ) / ( 0 - T1 ) ) ) / ( ( 0 - T1 ) ^ 2 );
    u0(3, 1) = 0;
else
    u0(1, 1) = ( 4 * Rx2 * ( pi ^ 2 ) * cos( ( 2 * pi * ( t - T1 ) ) / ( T1 - T2 ) ) ) / ( ( T1 - T2 ) ^ 2 );
    u0(2, 1) = - ( 16 * Ry2 * ( pi ^ 2 ) * sin( ( 4 * pi * ( t - T1 ) ) / ( T1 - T2 ) ) ) / ( ( T1 - T2 ) ^ 2 );
    u0(3, 1) = ( 16 * Rz2 * ( pi ^ 2 ) * sin( ( 4 * pi * ( t - T1 ) ) / ( T1 - T2 ) ) ) / ( ( T1 - T2 ) ^ 2 );
end

== matlab function sim_dist_pos_obs_paper/combine sigma_v ==
  data: sigma_v_1 input; sigma_v_2 input; sigma_v_3 input; sigma_v_4 input; sigma_v_5 input; sigma_v_vec output
function sigma_v_vec  = fcn(sigma_v_1, sigma_v_2, sigma_v_3, sigma_v_4, sigma_v_5)
%%%% 合并虚拟速度控制量sigma_v
sigma_v_vec = [sigma_v_1(:), sigma_v_2(:), sigma_v_3(:), sigma_v_4(:), sigma_v_5(:)];

== matlab function sim_dist_pos_obs_paper/cal combine sigma_bar_v ==
  data: eta_i_vec input; sigma_v_vec input; sigma_bar_v_vec output
function sigma_bar_v_vec = fcn(eta_i_vec, sigma_v_vec)
%%%% 计算虚拟速度追踪误差sigma_bar_v
sigma_bar_v_vec = zeros(3,5);
for iiuav = 1:5
    sigma_bar_v_vec(:,iiuav) = eta_i_vec(:,iiuav) - sigma_v_vec(:,iiuav);
end

== matlab function sim_dist_pos_obs_paper/cal differentiator d_sigma_bar_v_hat agent 1/cal differentiator ==
  data: c1 input; d_sigma_bar_v_hat output; d_dsigma_bar_v_hat output; d_d2sigma_bar_v_hat output; c2 input; c3 input; chi_t input; sigma_bar_v_sig_1 input; sigma_bar_v_sig_2 input; sigma_bar_v_sig_3 input; sigma_bar_v_sig_4 input; sigma_bar_v_sig_5 input; sigma_bar_v_sig_6 input; d_sigma_bar_v_hat input; d2_sigma_bar_v_hat input
function [d_sigma_bar_v_hat, d_dsigma_bar_v_hat, d_d2sigma_bar_v_hat] = fcn(c1, c2, c3, chi_t, sigma_bar_v_sig_1, sigma_bar_v_sig_2, sigma_bar_v_sig_3, ...
                                                                                                                                                sigma_bar_v_sig_4, sigma_bar_v_sig_5, sigma_bar_v_sig_6, d_sigma_bar_v_hat, d2_sigma_bar_v_hat)
d_d2sigma_bar_v_hat = -chi_t .* c1 * sigma_bar_v_sig_1(:) - (1 - chi_t) .* c1 * sigma_bar_v_sig_2(:);
d_dsigma_bar_v_hat = -chi_t .* c2 * sigma_bar_v_sig_3(:) - (1 - chi_t) .* c2 * sigma_bar_v_sig_4(:) + d2_sigma_bar_v_hat(:);
d_sigma_bar_v_hat = -chi_t .* c3 * sigma_bar_v_sig_5(:) - (1 - chi_t) .* c3 * sigma_bar_v_sig_6(:) + d_sigma_bar_v_hat(:);

== matlab function sim_dist_pos_obs_paper/cal differentiator d_sigma_bar_v_hat agent 1/cal sig ==
  data: x input; z output; y input
function z = fcn(x, y)
z = x(:) .* sign(y(:));

== matlab function sim_dist_pos_obs_paper/cal differentiator d_sigma_bar_v_hat agent 1/cal sig1 ==
  data: x input; z output; y input
function z = fcn(x, y)
z = x(:) .* sign(y(:));

== matlab function sim_dist_pos_obs_paper/cal differentiator d_sigma_bar_v_hat agent 1/cal sig2 ==
  data: x input; z output; y input
function z = fcn(x, y)
z = x(:) .* sign(y(:));

== matlab function sim_dist_pos_obs_paper/cal differentiator d_sigma_bar_v_hat agent 1/cal sig3 ==
  data: x input; z output; y input
function z = fcn(x, y)
z = x(:) .* sign(y(:));

== matlab function sim_dist_pos_obs_paper/cal differentiator d_sigma_bar_v_hat agent 1/cal sig4 ==
  data: x input; z output; y input
function z = fcn(x, y)
z = x(:) .* sign(y(:));

== matlab function sim_dist_pos_obs_paper/cal differentiator d_sigma_bar_v_hat agent 1/cal sig5 ==
  data: x input; z output; y input
function z = fcn(x, y)
z = x(:) .* sign(y(:));

== matlab function sim_dist_pos_obs_paper/cal differentiator d_sigma_bar_v_hat agent 1/choose sigma_bar_v ==
  data: x input; y output
function y = fcn(x)
iiuav = 1;
y = x(:,iiuav);

== matlab function sim_dist_pos_obs_paper/cal differentiator d_sigma_bar_v_hat agent 1/trans to column20 ==
  data: x input; y output
function y = fcn(x)
y = x(:);

== matlab function sim_dist_pos_obs_paper/cal differentiator d_sigma_bar_v_hat agent 1/trans to column21 ==
  data: x input; y output
function y = fcn(x)
y = x(:);

== matlab function sim_dist_pos_obs_paper/cal differentiator d_sigma_bar_v_hat agent 1/trans to column22 ==
  data: x input; y output
function y = fcn(x)
y = x(:);

== matlab function sim_dist_pos_obs_paper/cal differentiator d_sigma_bar_v_hat agent 1/trans to column23 ==
  data: x input; y output
function y = fcn(x)
y = x(:);

== matlab function sim_dist_pos_obs_paper/cal differentiator d_sigma_bar_v_hat agent 1/trans to column24 ==
  data: x input; y output
function y = fcn(x)
y = x(:);

== matlab function sim_dist_pos_obs_paper/cal differentiator d_sigma_bar_v_hat agent 1/trans to column25 ==
  data: x input; y output
function y = fcn(x)
y = x(:);

== matlab function sim_dist_pos_obs_paper/cal differentiator d_sigma_bar_v_hat agent 2/cal differentiator ==
  data: c1 input; d_sigma_bar_v_hat output; d_dsigma_bar_v_hat output; d_d2sigma_bar_v_hat output; c2 input; c3 input; chi_t input; sigma_bar_v_sig_1 input; sigma_bar_v_sig_2 input; sigma_bar_v_sig_3 input; sigma_bar_v_sig_4 input; sigma_bar_v_sig_5 input; sigma_bar_v_sig_6 input; d_sigma_bar_v_hat input; d2_sigma_bar_v_hat input
function [d_sigma_bar_v_hat, d_dsigma_bar_v_hat, d_d2sigma_bar_v_hat] = fcn(c1, c2, c3, chi_t, sigma_bar_v_sig_1, sigma_bar_v_sig_2, sigma_bar_v_sig_3, ...
                                                                                                                                                sigma_bar_v_sig_4, sigma_bar_v_sig_5, sigma_bar_v_sig_6, d_sigma_bar_v_hat, d2_sigma_bar_v_hat)
d_d2sigma_bar_v_hat = -chi_t .* c1 * sigma_bar_v_sig_1(:) - (1 - chi_t) .* c1 * sigma_bar_v_sig_2(:);
d_dsigma_bar_v_hat = -chi_t .* c2 * sigma_bar_v_sig_3(:) - (1 - chi_t) .* c2 * sigma_bar_v_sig_4(:) + d2_sigma_bar_v_hat(:);
d_sigma_bar_v_hat = -chi_t .* c3 * sigma_bar_v_sig_5(:) - (1 - chi_t) .* c3 * sigma_bar_v_sig_6(:) + d_sigma_bar_v_hat(:);

== matlab function sim_dist_pos_obs_paper/generate translational disturbance agent 5 ==
  data: dp_aa_t input; dp_ff_t input; dp_phi_t input; dp_5 output; t input
function dp_5 = fcn(dp_aa_t, dp_ff_t, dp_phi_t, t)
%%%% 平移动力学方程中的扰动项设置
epsil_t = zeros(3, 1);

for kk = 1:5
    epsil_t = epsil_t + dp_aa_t(:, kk) .* sin( 2 * pi * dp_ff_t(:, kk) * t + dp_phi_t(:, kk) );
end

dp_5 = [ epsil_t(1) + 1.6 * sin( 0.2 * t ) + 2.0 * cos( 0.3 * t ) + 1.4 * sin( 0.5 * t ) ...
                + 4 * exp( -0.1 * t ) * sin( 0.5 * t ) + 3 / ( 1 + exp( -0.2 * ( t - 15 ) ) ); ...
                epsil_t(2) + 1.2 * sin( 0.1 * t ) + 3 * cos( 0.2 * t ) + 0.8 * sin( 0.4 * t ) ...
                + 2 * exp( -0.15 * t ) * cos( 0.6 * t ) + 3 / ( 1 + exp( -0.3 * ( t - 25 ) ) ); ...
                epsil_t(3) + 1.8 * sin( 0.1 * t ) + 1.6 * sin( 0.2 * t ) + 1.6 * cos( 0.3 * t ) ...
                + 4 * exp( -0.05 * t ) * sin( 0.4 * t + pi / 4 ) + 3 / ( 1 + exp( -0.5 * ( t - 20 ) ) ) ];

== matlab function sim_dist_pos_obs_paper/cal Rei ==
  data: Rei output; Qei input
function Rei = fcn(Qei)
%%%% 使用罗德里格公式由四元数Qei求解Rei
Rei = zeros(3,3,5);
for iuav = 1:5
    thetaei_tmp = Qei(1,iuav);
    qei_tmp = Qei(2:4,iuav);
    Rei(:,:,iuav) = ((thetaei_tmp^2) - (qei_tmp')*qei_tmp) * eye(3,3) ...
                            + 2 * qei_tmp * (qei_tmp') ...
                            - 2 * thetaei_tmp * cal_askew_mat(qei_tmp);
end

end

== matlab function sim_dist_pos_obs_paper/cal differentiator d_sigma_bar_v_hat agent 2/cal sig ==
  data: x input; z output; y input
function z = fcn(x, y)
z = x(:) .* sign(y(:));

== matlab function sim_dist_pos_obs_paper/cal differentiator d_sigma_bar_v_hat agent 2/cal sig1 ==
  data: x input; z output; y input
function z = fcn(x, y)
z = x(:) .* sign(y(:));

== matlab function sim_dist_pos_obs_paper/cal differentiator d_sigma_bar_v_hat agent 2/cal sig2 ==
  data: x input; z output; y input
function z = fcn(x, y)
z = x(:) .* sign(y(:));

== matlab function sim_dist_pos_obs_paper/cal differentiator d_sigma_bar_v_hat agent 2/cal sig3 ==
  data: x input; z output; y input
function z = fcn(x, y)
z = x(:) .* sign(y(:));

== matlab function sim_dist_pos_obs_paper/cal differentiator d_sigma_bar_v_hat agent 2/cal sig4 ==
  data: x input; z output; y input
function z = fcn(x, y)
z = x(:) .* sign(y(:));

== matlab function sim_dist_pos_obs_paper/cal differentiator d_sigma_bar_v_hat agent 2/cal sig5 ==
  data: x input; z output; y input
function z = fcn(x, y)
z = x(:) .* sign(y(:));

== matlab function sim_dist_pos_obs_paper/cal differentiator d_sigma_bar_v_hat agent 2/choose sigma_bar_v ==
  data: x input; y output
function y = fcn(x)
iiuav = 2;
y = x(:,iiuav);

== matlab function sim_dist_pos_obs_paper/cal differentiator d_sigma_bar_v_hat agent 2/trans to column20 ==
  data: x input; y output
function y = fcn(x)
y = x(:);

== matlab function sim_dist_pos_obs_paper/cal differentiator d_sigma_bar_v_hat agent 2/trans to column21 ==
  data: x input; y output
function y = fcn(x)
y = x(:);

== matlab function sim_dist_pos_obs_paper/cal differentiator d_sigma_bar_v_hat agent 2/trans to column22 ==
  data: x input; y output
function y = fcn(x)
y = x(:);
